simulink model "pendulum_sim"  (R2020a)
settings: Solver=VariableStepAuto  StartTime=0.0  StopTime=Tf  RelTol=1e-3
undefined symbols (not defined in the file): disable_noise, Ts
settings Model: Creator=Valentina  LastModifiedBy=giaco

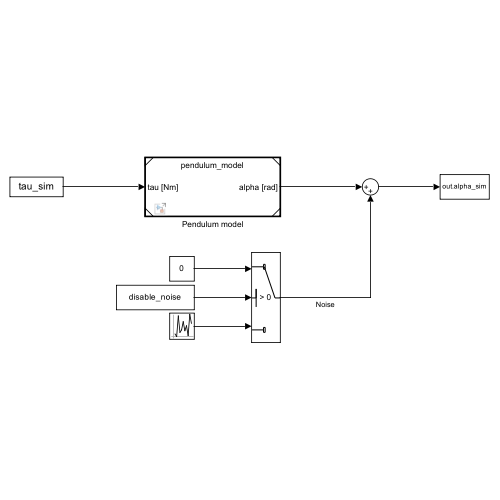
[thumbnail: Simulink's stored preview of the top-level diagram]
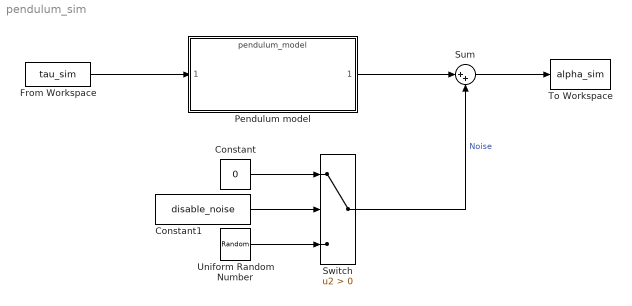
== system pendulum_sim ==
  Constant : Constant  Value=0
  Constant1 : Constant  Value=disable_noise  OutDataTypeStr=boolean
  From Workspace : FromWorkspace  VariableName=tau_sim  SampleTime=Ts
  Pendulum model : ModelReference  ModelNameDialog=pendulum_model.slx  SimulationMode=Normal  ModelReferenceVersion=6.2
  Sum : Sum  Inputs=|++
  Switch : Switch  Criteria=u2 > Threshold
  To Workspace : ToWorkspace  VariableName=alpha_sim  SampleTime=Ts
  Uniform Random Number : UniformRandomNumber  Minimum=-pi/180  Maximum=pi/180  Seed=414  SampleTime=Ts
  wires:
  From Workspace/1 -> Pendulum model/1
  Constant/1 -> Switch/1
  Switch/1 -> Sum/2  "Noise"
  Pendulum model/1 -> Sum/1
  Sum/1 -> To Workspace/1
  Uniform Random Number/1 -> Switch/3
  Constant1/1 -> Switch/2
